simulink model "gan_hemt_digital_twin"  (R2026a)
settings: Solver=ode3  StartTime=0  StopTime=1e-5  FixedStep=1e-09  MaxStep=1e-09
settings Model: Creator=aSh..!  LastModifiedBy=aSh..!

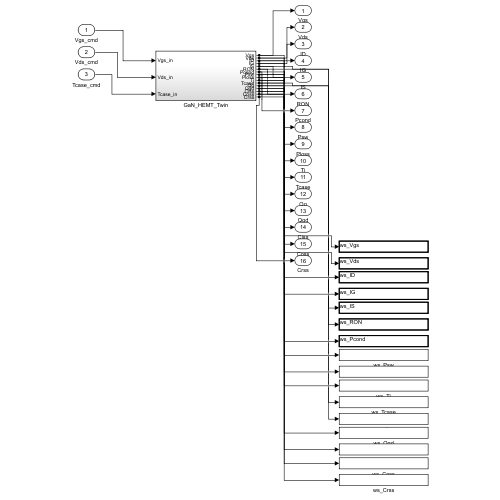
[thumbnail: Simulink's stored preview of the top-level diagram]
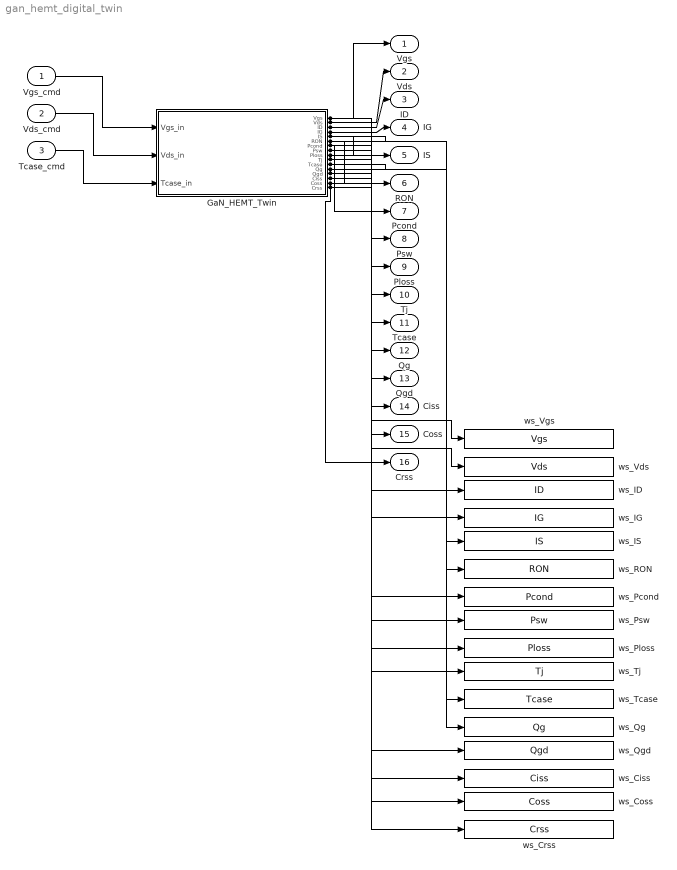
== system gan_hemt_digital_twin ==
  Vgs_cmd : Inport  PortDimensions=1
  Vds_cmd : Inport  Port=2  PortDimensions=1
  Tcase_cmd : Inport  Port=3  PortDimensions=1
  GaN_HEMT_Twin : Subsystem
  ws_Ciss : ToWorkspace  VariableName=Ciss  SampleTime=-1
  ws_Coss : ToWorkspace  VariableName=Coss  SampleTime=-1
  ws_Crss : ToWorkspace  VariableName=Crss  SampleTime=-1
  ws_ID : ToWorkspace  VariableName=ID  SampleTime=-1
  ws_IG : ToWorkspace  VariableName=IG  SampleTime=-1
  ws_IS : ToWorkspace  VariableName=IS  SampleTime=-1
  ws_Pcond : ToWorkspace  VariableName=Pcond  SampleTime=-1
  ws_Ploss : ToWorkspace  VariableName=Ploss  SampleTime=-1
  ws_Psw : ToWorkspace  VariableName=Psw  SampleTime=-1
  ws_Qg : ToWorkspace  VariableName=Qg  SampleTime=-1
  ws_Qgd : ToWorkspace  VariableName=Qgd  SampleTime=-1
  ws_RON : ToWorkspace  VariableName=RON  SampleTime=-1
  ws_Tcase : ToWorkspace  VariableName=Tcase  SampleTime=-1
  ws_Tj : ToWorkspace  VariableName=Tj  SampleTime=-1
  ws_Vds : ToWorkspace  VariableName=Vds  SampleTime=-1
  ws_Vgs : ToWorkspace  VariableName=Vgs  SampleTime=-1
  Vgs : Outport
  Vds : Outport  Port=2
  ID : Outport  Port=3
  IG : Outport  Port=4
  IS : Outport  Port=5
  RON : Outport  Port=6
  Pcond : Outport  Port=7
  Psw : Outport  Port=8
  Ploss : Outport  Port=9
  Tj : Outport  Port=10
  Tcase : Outport  Port=11
  Qg : Outport  Port=12
  Qgd : Outport  Port=13
  Ciss : Outport  Port=14
  Coss : Outport  Port=15
  Crss : Outport  Port=16
  wires:
  Vgs_cmd/1 -> GaN_HEMT_Twin/1(Vgs_in)
  Vds_cmd/1 -> GaN_HEMT_Twin/2(Vds_in)
  Tcase_cmd/1 -> GaN_HEMT_Twin/3(Tcase_in)
  GaN_HEMT_Twin/1(Vgs) -> Vgs/1, ws_Vgs/1
  GaN_HEMT_Twin/2(Vds) -> Vds/1, ws_Vds/1
  GaN_HEMT_Twin/3(ID) -> ID/1, ws_ID/1
  GaN_HEMT_Twin/4(IG) -> IG/1, ws_IG/1
  GaN_HEMT_Twin/5(IS) -> IS/1, ws_IS/1
  GaN_HEMT_Twin/6(RON) -> RON/1, ws_RON/1
  GaN_HEMT_Twin/7(Pcond) -> Pcond/1, ws_Pcond/1
  GaN_HEMT_Twin/8(Psw) -> Psw/1, ws_Psw/1
  GaN_HEMT_Twin/9(Ploss) -> Ploss/1, ws_Ploss/1
  GaN_HEMT_Twin/10(Tj) -> Tj/1, ws_Tj/1
  GaN_HEMT_Twin/11(Tcase) -> Tcase/1, ws_Tcase/1
  GaN_HEMT_Twin/12(Qg) -> Qg/1, ws_Qg/1
  GaN_HEMT_Twin/13(Qgd) -> Qgd/1, ws_Qgd/1
  GaN_HEMT_Twin/14(Ciss) -> Ciss/1, ws_Ciss/1
  GaN_HEMT_Twin/15(Coss) -> Coss/1, ws_Coss/1
  GaN_HEMT_Twin/16(Crss) -> Crss/1, ws_Crss/1

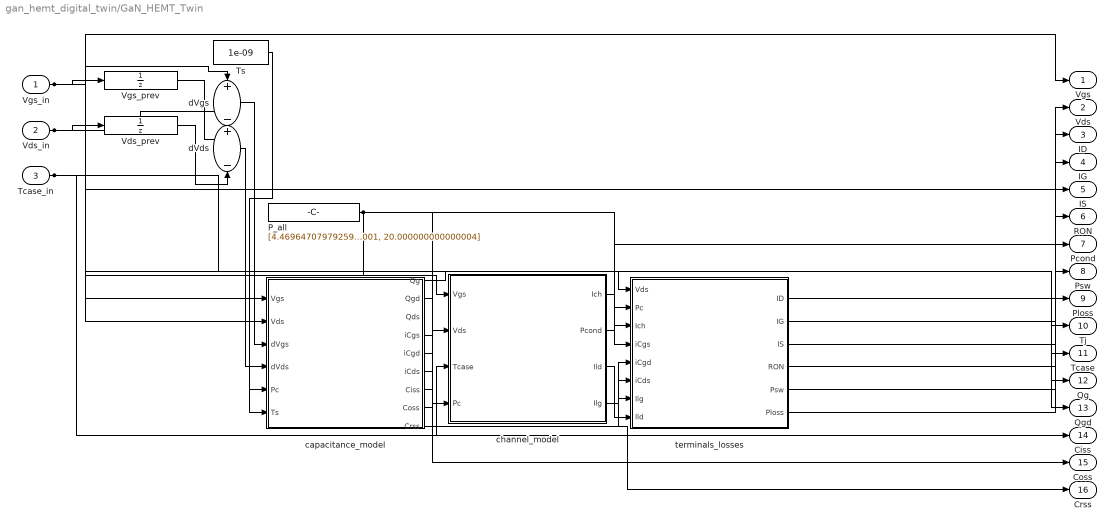
== system gan_hemt_digital_twin/GaN_HEMT_Twin ==
  Vgs_in : Inport  PortDimensions=1
  Vds_in : Inport  Port=2  PortDimensions=1
  Tcase_in : Inport  Port=3  PortDimensions=1
  P_all : Constant  Value=[4.4696470797925946e-10, 3.3297138138527536, 7.0629414643249729e-09, 14.586648712891728, 4.7820000000000002e-09, 1.5866498795014214, 1.1000000000000001, -4, 161.91709844559585, 0.050000000000000003, 1.6630271007940307, 100, 3.9999999999999998e-06, 150, 1.9999999999999999e-06, 6, 0.5, 15.000000000000002, 100, 25, 0.10000000000000001, 20.000000000000004]
  Ts : Constant  Value=1e-09
  Vds_prev : UnitDelay  SampleTime=1e-09
  Vgs_prev : UnitDelay  SampleTime=1e-09
  capacitance_model : MATLAB Function  TreatAsAtomicUnit=on
  channel_model : MATLAB Function  TreatAsAtomicUnit=on
  dVds : Sum  Inputs=+-
  dVgs : Sum  Inputs=+-
  terminals_losses : MATLAB Function  TreatAsAtomicUnit=on
  Vgs : Outport
  Vds : Outport  Port=2
  ID : Outport  Port=3
  IG : Outport  Port=4
  IS : Outport  Port=5
  RON : Outport  Port=6
  Pcond : Outport  Port=7
  Psw : Outport  Port=8
  Ploss : Outport  Port=9
  Tj : Outport  Port=10
  Tcase : Outport  Port=11
  Qg : Outport  Port=12
  Qgd : Outport  Port=13
  Ciss : Outport  Port=14
  Coss : Outport  Port=15
  Crss : Outport  Port=16
  wires:
  ? -> ?
  Vgs_in/1 -> Vgs_prev/1, dVgs/1, capacitance_model/1(Vgs), channel_model/1(Vgs), Vgs/1
  Vgs_prev/1 -> dVgs/2
  Vds_in/1 -> Vds_prev/1, dVds/1, capacitance_model/2(Vds), channel_model/2(Vds), terminals_losses/1(Vds), Vds/1
  Vds_prev/1 -> dVds/2
  dVgs/1 -> capacitance_model/3(dVgs)
  dVds/1 -> capacitance_model/4(dVds)
  P_all/1 -> capacitance_model/5(Pc), channel_model/4(Pc), terminals_losses/2(Pc)
  Ts/1 -> capacitance_model/6(Ts)
  Tcase_in/1 -> channel_model/3(Tcase), Tj/1, Tcase/1
  channel_model/1(Ich) -> terminals_losses/3(Ich)
  capacitance_model/4(iCgs) -> terminals_losses/4(iCgs)
  capacitance_model/5(iCgd) -> terminals_losses/5(iCgd)
  capacitance_model/6(iCds) -> terminals_losses/6(iCds)
  channel_model/4(Ilg) -> terminals_losses/7(Ilg)
  channel_model/3(Ild) -> terminals_losses/8(Ild)
  terminals_losses/1(ID) -> ID/1
  terminals_losses/2(IG) -> IG/1
  terminals_losses/3(IS) -> IS/1
  terminals_losses/4(RON) -> RON/1
  channel_model/2(Pcond) -> Pcond/1
  terminals_losses/5(Psw) -> Psw/1
  terminals_losses/6(Ploss) -> Ploss/1
  capacitance_model/1(Qg) -> Qg/1
  capacitance_model/2(Qgd) -> Qgd/1
  capacitance_model/7(Ciss) -> Ciss/1
  capacitance_model/8(Coss) -> Coss/1
  capacitance_model/9(Crss) -> Crss/1

== matlab function gan_hemt_digital_twin/GaN_HEMT_Twin/channel_model ==
  data: Vgs input; Ich output; Vds input; Tcase input; Pc input; Pcond output; Ild output; Ilg output
function [Ich,Pcond,Ild,Ilg] = fcn(Vgs,Vds,Tcase,Pc)
%#codegen
% Pc is the flat parameter vector; see p.model.vector_names.
k = Pc(9); vth = Pc(7); vsmooth = Pc(10); vdsat_max = Pc(11); va = Pc(12);
idss = Pc(13); vdss_ref = Pc(14); igss = Pc(15); vgs_max = Pc(16);
vigs_iso = Pc(17); leak_ratio = Pc(18); leak_span = Pc(19); tnom = Pc(20);
igss_ratio = Pc(22);

Vov = Vgs - vth;
Vc  = 0.5 * Vov .* (1 + tanh(Vov ./ (2*vsmooth)));
Vda = abs(Vds);
Vdsat = min(max(Vc,0), vdsat_max);
Vdc  = min(Vda, Vdsat);
Ich  = sign(Vds) .* k .* (Vc .* Vdc - 0.5*Vdc.^2) .* (1 + Vda ./ va);
Pcond = Vds .* Ich;

% Leakage magnitudes are anchored to the datasheet maxima; the temperature
% ratio comes from the two printed IDSS points.
tf  = leak_ratio .^ ((Tcase - tnom) ./ leak_span);
tf_exp = (Tcase - tnom) ./ leak_span;
Ild = idss .* (min(Vda, vdss_ref) ./ vdss_ref).^0.5 .* tf;
Ilg = -igss .* tanh(-Vgs ./ vigs_iso) ./ tanh(-vgs_max ./ vigs_iso) .* (igss_ratio .^ tf_exp);
end

== matlab function gan_hemt_digital_twin/GaN_HEMT_Twin/capacitance_model ==
  data: Vgs input; Qg output; Vds input; dVgs input; dVds input; Pc input; Ts input; Qgd output; Qds output; iCgs output; iCgd output; iCds output; Ciss output; Coss output; Crss output
function [Qg,Qgd,Qds,iCgs,iCgd,iCds,Ciss,Coss,Crss] = fcn(Vgs,Vds,dVgs,dVds,Pc,Ts)
%#codegen
% Pc is the flat parameter vector; see p.model.vector_names.
cgd0 = Pc(1); vjg = Pc(2); coss0 = Pc(3); vjc = Pc(4);
cgs0 = Pc(5); vgsc = Pc(6); vth = Pc(7); vgs_min = Pc(8);

vg  = max(Vgs, vgs_min);
va  = abs(Vds);
sgn = sign(Vds);

% Depletion capacitances: C(V) = C0 / (1 + |V| / Vj).
Cgd  = cgd0 ./ (1 + va ./ vjg);
Coss = coss0 ./ (1 + va ./ vjc);
Cds  = Coss - Cgd;
Cgs  = cgs0 ./ (1 + max(vg,0) ./ vgsc);
Ciss = Cgs + 2*Cgd;
Crss = Cgd;

% Integrated charge forms of the same depletion curves.
qgd_d  = cgd0  .* vjg  .* log(1 + va ./ vjg);
qoss_d = coss0 .* vjc .* log(1 + va ./ vjc);
qgs_g  = cgs0 .* vgsc .* log(1 + max(vg,0) ./ vgsc);

% Above threshold the Miller charge acquires a gate-referred term.
Vc  = max(Vgs - vth, 0);
Qgd = qgd_d + Cgd .* Vc;
Qgs = qgs_g;
Qds = qoss_d - qgd_d;
Qg  = Qgs + Qgd;

dvgs_dt = dVgs ./ Ts;
dvds_dt = dVds ./ Ts;
iCgd = Cgd .* sgn .* dvds_dt + Cgd .* double(Vgs > vth) .* dvgs_dt;
iCds = Cds .* sgn .* dvds_dt;
iCgs = Cgs .* dvgs_dt;
end

== matlab function gan_hemt_digital_twin/GaN_HEMT_Twin/terminals_losses ==
  data: Vds input; ID output; Pc input; Ich input; iCgs input; iCgd input; iCds input; Ilg input; Ild input; IG output; IS output; RON output; Psw output; Ploss output
function [ID,IG,IS,RON,Psw,Ploss] = fcn(Vds,Pc,Ich,iCgs,iCgd,iCds,Ilg,Ild)
%#codegen
ron_ithresh = Pc(21);

ID = Ich + iCgd + iCds + Ild;
IG = iCgs + iCgd + Ilg;
IS = -(ID + IG);

RON = NaN(size(ID));
mask = ID > ron_ithresh;
RON(mask) = Vds(mask) ./ ID(mask);

Psw   = Vds .* abs(iCgd);
Ploss = Vds .* Ich + Psw;
end
